simulink subsystem "Vehicle1D_Custom_refsub"  (R2026a)
settings: Solver=VariableStepAuto
PreLoadFcn:
  | defineBus_Rotational
libraries: nesl_utility x5, fl_lib x1
settings Model: Creator=isaacito  LastModifiedBy=isaacito
settings SimscapeCC: SimscapeNominalValues="[{\"value\":\"1\",\"unit\":\"A\"},{\"value\":\"1\",\"unit\":\"bar\"},{\"value\":\"1\",\"unit\":\"cm^2\"},{\"value\":\"1\",\"unit\":\"cm^3/s\"},{\"value\":\"1\",\"unit\":\"kJ/kg\"},{\"value\":\"1\",\"unit\":\"kW\"},{\"value\":\"1\",\"unit\":\"l\"},{\"value\":\"1\",\"unit\":\"N\"},{\"value\":\"1\",\"unit\":\"N*m\"},{\"value\":\"1\",\"unit\":\"V\"}]"  SimscapeLogType=none  SimscapeLogDataHistory=5000.0

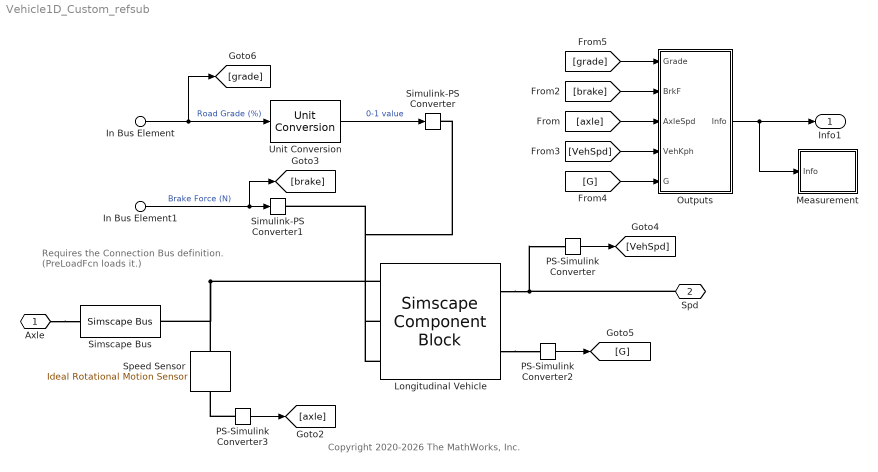
== system Vehicle1D_Custom_refsub ==
  note: Requires the Connection Bus definition.
      | (PreLoadFcn loads it.)
  note: Copyright 2020-2026 The MathWorks, Inc.
  In Bus Element : Inport  PortName=Inputs  Element=RoadGrade
      settings: AttributesFormatString=%<Unit>
  In Bus Element1 : Inport  PortName=Inputs  Element=BrakeForce
      settings: AttributesFormatString=%<Unit>
  Longitudinal Vehicle : SimscapeComponentBlock  SourceFile=Vehicle1D_Custom  ComponentPath=Vehicle1D_Custom  ComponentVariants="[\"Vehicle1D_Custom\"]"  ComponentVariantNames="[\"Vehicle1D_Custom\"]"  ClassName=Vehicle1D_Custom  SchemaVersion=1  grav=9.81 m/s^2  M_e=vehicle.mass_kg kg  R_tire=vehicle.tireRollingRadius_m m  A_rl=vehicle.roadLoadA_N N  B_rl=vehicle.roadLoadB_N_per_kph N*hr/km  C_rl=vehicle.roadLoadC_N_per_kph2 N*hr^2/km^2  V_1=smoothing.vehicle_speedThreshold_kph km/hr  w_1=smoothing.vehicle_axleSpeedThreshold_rpm rpm  V_x_specify=on  V_x_priority=High  V_x=initial.vehicle_speed_kph km/hr  V_x_nominal_specify=off  V_x_nominal_value=1  V_x_nominal_unit=km/hr
      settings: AttributesFormatString=%<V_x>  CopyFcn=simscape.sscblock.internal.componentBlockCallback(gcbh,'COPY')  PreCopyFcn=simscape.sscblock.internal.componentBlockCallback(gcbh,'PRECOPY')  PreDeleteFcn=simscape.sscblock.internal.componentBlockCallback(gcbh,'PREDELETE')  LogSimulationData=on
      mask Type: Custom Longitudinal Vehicle
  Measurement : Subsystem
  Outputs : Subsystem
  PS-Simulink Converter : nesl_utility/PS-Simulink Converter  PhysicalDomain=network_engine_domain  SubClassName=ps_output  LeftPortType=input  RightPortType=output  PseudoPeriodic=off  Frequencies=[]  VectorFormat=1-D array  Unit=km/hr  AffineConversion=off
  PS-Simulink Converter2 : nesl_utility/PS-Simulink Converter  PhysicalDomain=network_engine_domain  SubClassName=ps_output  LeftPortType=input  RightPortType=output  PseudoPeriodic=off  Frequencies=[]  VectorFormat=1-D array  Unit=1  AffineConversion=off
  PS-Simulink Converter3 : nesl_utility/PS-Simulink Converter  PhysicalDomain=network_engine_domain  SubClassName=ps_output  LeftPortType=input  RightPortType=output  PseudoPeriodic=off  Frequencies=[]  VectorFormat=1-D array  Unit=rpm  AffineConversion=off
  Simscape Bus : SimscapeBus  HierarchyStrings=AngSpd  ConnectionType=Bus: Bus_Rotational
      settings: AttributesFormatString=%<ConnectionType>
  Simulink-PS Converter : nesl_utility/Simulink-PS Converter  PhysicalDomain=network_engine_domain  SubClassName=ps_input  LeftPortType=input  RightPortType=output  PseudoPeriodic=off  Frequencies=[]  NoiseDistribution=none  NoiseParameters=[]  Unit=1  AffineConversion=off  FilteringAndDerivatives=filter  SimscapeFilterOrder=1  InputFilterTimeConstant=0.001  UdotUserProvided=0
  Simulink-PS Converter1 : nesl_utility/Simulink-PS Converter  PhysicalDomain=network_engine_domain  SubClassName=ps_input  LeftPortType=input  RightPortType=output  PseudoPeriodic=off  Frequencies=[]  NoiseDistribution=none  NoiseParameters=[]  Unit=N  AffineConversion=off  FilteringAndDerivatives=filter  SimscapeFilterOrder=1  InputFilterTimeConstant=0.001  UdotUserProvided=0
  Speed Sensor : fl_lib/Mechanical/Mechanical Sensors/Ideal Rotational Motion Sensor  reference=foundation.enum.MeasurementReference.absolute  acceleration_port=false  velocity_port=true  position_port=false  wrap_angle=simscape.enum.onoff.off  offset=0 rad
  Unit Conversion : UnitConversion  OutputType=Inherit: Inherit via back propagation
  Axle : PMIOPort  Side=Left
  Spd : PMIOPort  Port=2  Side=Right
  Info1 : Outport
  wires:
  PS-Simulink Converter/1 -> [VehSpd]
  PS-Simulink Converter2/1 -> [G]
  In Bus Element/1 -> Unit Conversion/1, [grade]  "Road Grade (%)"
  In Bus Element1/1 -> [brake], Simulink-PS Converter1/1  "Brake Force (N)"
  Unit Conversion/1 -> Simulink-PS Converter/1  "0-1 value"
  PS-Simulink Converter3/1 -> [axle]
  Outputs/1(Info) -> Measurement/1(Info), Info1/1
  [grade] -> Outputs/1(Grade)
  [brake] -> Outputs/2(BrkF)
  [axle] -> Outputs/3(AxleSpd)
  [VehSpd] -> Outputs/4(VehKph)
  [G] -> Outputs/5(G)
  connections:
  Longitudinal Vehicle/RConn1 -- Spd/RConn1 -- PS-Simulink Converter/LConn1
  Longitudinal Vehicle/LConn1 -- Speed Sensor/LConn1 -- Simscape Bus/LConn1
  Longitudinal Vehicle/RConn2 -- PS-Simulink Converter2/LConn1
  Longitudinal Vehicle/LConn3 -- Simulink-PS Converter/RConn1
  Longitudinal Vehicle/LConn2 -- Simulink-PS Converter1/RConn1
  Axle/RConn1 -- Simscape Bus/RConn1
  PS-Simulink Converter3/LConn1 -- Speed Sensor/RConn1

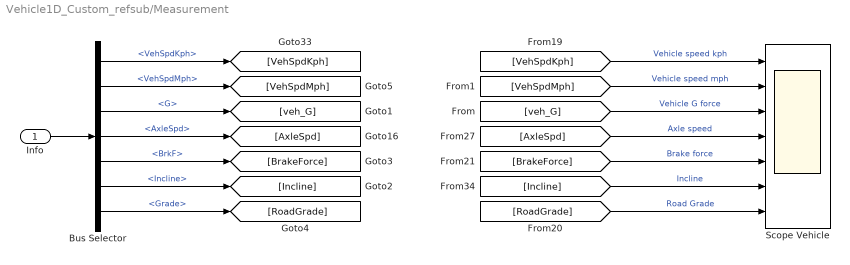
== system Vehicle1D_Custom_refsub/Measurement ==
  Info : Inport
  Bus Selector : BusSelector  OutputSignals=VehSpdKph,VehSpdMph,G,AxleSpd,BrkF,Incline,Grade
  Scope Vehicle : Scope  NumInputPorts=7
      settings: ActiveDisplayYMinimum=-12.00926  ActiveDisplayYMaximum=102.7511
  wires:
  Bus Selector/6 -> [Incline]  "<Incline>"
  Bus Selector/7 -> [RoadGrade]  "<Grade>"
  Bus Selector/5 -> [BrakeForce]  "<BrkF>"
  Bus Selector/4 -> [AxleSpd]  "<AxleSpd>"
  Bus Selector/3 -> [veh_G]  "<G>"
  Bus Selector/2 -> [VehSpdMph]  "<VehSpdMph>"
  Bus Selector/1 -> [VehSpdKph]  "<VehSpdKph>"
  Info/1 -> Bus Selector/1
  [VehSpdMph] -> Scope Vehicle/2  "Vehicle speed mph"
  [RoadGrade] -> Scope Vehicle/7  "Road Grade"
  [Incline] -> Scope Vehicle/6  "Incline"
  [BrakeForce] -> Scope Vehicle/5  "Brake force"
  [AxleSpd] -> Scope Vehicle/4  "Axle speed"
  [veh_G] -> Scope Vehicle/3  "Vehicle G force"
  [VehSpdKph] -> Scope Vehicle/1  "Vehicle speed kph"

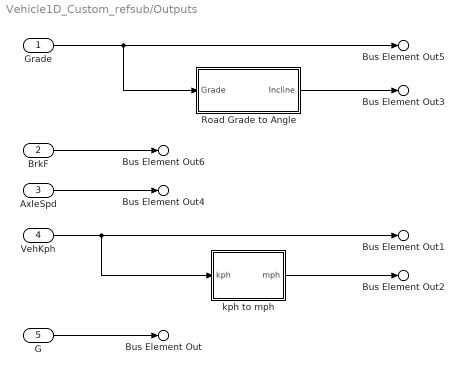
== system Vehicle1D_Custom_refsub/Outputs ==
  Grade : Inport  Unit=%
      settings: AttributesFormatString=%<Unit>
  BrkF : Inport  Port=2  Unit=N
      settings: AttributesFormatString=%<Unit>
  AxleSpd : Inport  Port=3  Unit=rpm
      settings: AttributesFormatString=%<Unit>
  VehKph : Inport  Port=4  Unit=km/hr
      settings: AttributesFormatString=%<Unit>
  G : Inport  Port=5  Unit=1
      settings: AttributesFormatString=%<Unit>
  Road Grade to Angle : Subsystem
  kph to mph : Subsystem
  Bus Element Out : Outport  PortName=Info  Element=G
      settings: AttributesFormatString=%<Unit>
  Bus Element Out1 : Outport  PortName=Info  Element=VehSpdKph
      settings: AttributesFormatString=%<Unit>
  Bus Element Out2 : Outport  PortName=Info  Element=VehSpdMph
      settings: AttributesFormatString=%<Unit>
  Bus Element Out3 : Outport  PortName=Info  Element=Incline
      settings: AttributesFormatString=%<Unit>
  Bus Element Out4 : Outport  PortName=Info  Element=AxleSpd
      settings: AttributesFormatString=%<Unit>
  Bus Element Out5 : Outport  PortName=Info  Element=Grade
      settings: AttributesFormatString=%<Unit>
  Bus Element Out6 : Outport  PortName=Info  Element=BrkF
      settings: AttributesFormatString=%<Unit>
  wires:
  kph to mph/1(mph) -> Bus Element Out2/1
  Road Grade to Angle/1(Incline) -> Bus Element Out3/1
  Grade/1 -> Bus Element Out5/1, Road Grade to Angle/1(Grade)
  BrkF/1 -> Bus Element Out6/1
  G/1 -> Bus Element Out/1
  VehKph/1 -> Bus Element Out1/1, kph to mph/1(kph)
  AxleSpd/1 -> Bus Element Out4/1

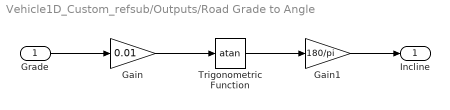
== system Vehicle1D_Custom_refsub/Outputs/Road Grade to Angle ==
  Grade : Inport  Unit=%
      settings: AttributesFormatString=%<Unit>
  Gain : Gain  Gain=0.01
  Gain1 : Gain  Gain=180/pi
  Trigonometric Function : Trigonometry  Operator=atan
  Incline : Outport  Unit=deg
      settings: AttributesFormatString=%<Unit>
  wires:
  Gain/1 -> Trigonometric Function/1
  Grade/1 -> Gain/1
  Trigonometric Function/1 -> Gain1/1
  Gain1/1 -> Incline/1

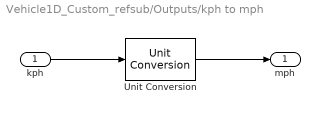
== system Vehicle1D_Custom_refsub/Outputs/kph to mph ==
  kph : Inport  Unit=km/h
  Unit Conversion : UnitConversion
  mph : Outport  Unit=mph
  wires:
  Unit Conversion/1 -> mph/1
  kph/1 -> Unit Conversion/1
